simulink model "PD"  (R2018b)
settings: Solver=VariableStepAuto  StartTime=0.0  StopTime=2  RelTol=1e-3
undefined symbols (not defined in the file): A, C
settings Model: Creator=bernardo  LastModifiedBy=bernardo

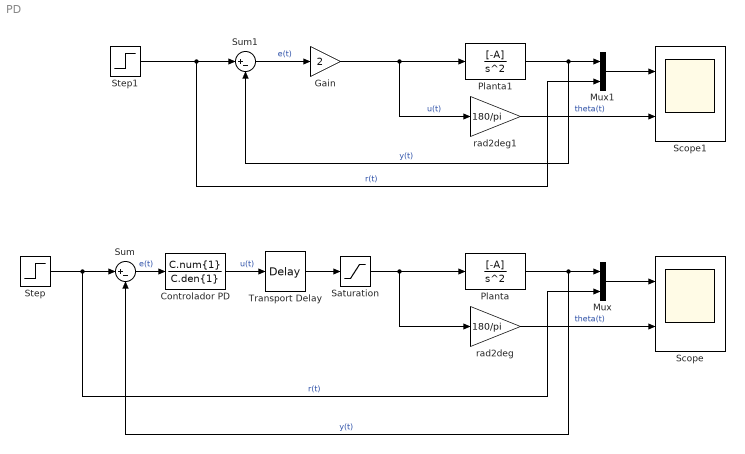
== system PD ==
  Controlador PD : TransferFcn  Numerator=C.num{1}  Denominator=C.den{1}
  Gain : Gain  Gain=2
  Mux : Mux  Inputs=2
  Mux1 : Mux  Inputs=2
  Planta : TransferFcn  Numerator=[-A]  Denominator=[1 0 0]
  Planta1 : TransferFcn  Numerator=[-A]  Denominator=[1 0 0]
  Saturation : Saturate  UpperLimit=50*pi/180  LowerLimit=-30*pi/180
  Scope : Scope  NumInputPorts=2
  Scope1 : Scope  NumInputPorts=2
  Step : Step  After=20  SampleTime=0.01
  Step1 : Step  Time=0.5  After=20  SampleTime=0.001
  Sum : Sum  Inputs=|+-
  Sum1 : Sum  Inputs=|+-
  Transport Delay : TransportDelay  DelayTime=0.05
  rad2deg : Gain  Gain=180/pi
  rad2deg1 : Gain  Gain=180/pi
  wires:
  Controlador PD/1 -> Transport Delay/1  "u(t)"
  Sum/1 -> Controlador PD/1  "e(t)"
  Planta/1 -> Mux/1, Sum/2  "y(t)"
  Step/1 -> Sum/1, Mux/2  "r(t)"
  Mux/1 -> Scope/1
  rad2deg/1 -> Scope/2  "theta(t)"
  Transport Delay/1 -> Saturation/1
  Saturation/1 -> Planta/1, rad2deg/1
  Sum1/1 -> Gain/1  "e(t)"
  Gain/1 -> Planta1/1, rad2deg1/1  "u(t)"
  Step1/1 -> Sum1/1, Mux1/2  "r(t)"
  Planta1/1 -> Mux1/1, Sum1/2  "y(t)"
  rad2deg1/1 -> Scope1/2  "theta(t)"
  Mux1/1 -> Scope1/1
